simulink model "zadatak2"  (R2013b)
settings: Solver=ode45  StartTime=0.0  StopTime=10.0  RelTol=1e-3
settings Model: Creator=KORISNIK  LastModifiedBy=KORISNIK

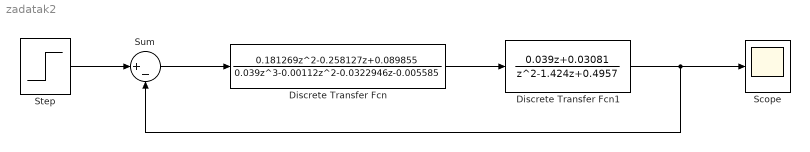
== system zadatak2 ==
  Discrete Transfer Fcn : DiscreteTransferFcn  Numerator=[0.181269 -0.258127 0.089855]  Denominator=[0.039 -0.00112 -0.0322946 -0.005585]  SampleTime=0.1
  Discrete Transfer Fcn1 : DiscreteTransferFcn  Numerator=[0.039 0.03081]  Denominator=[1 -1.424 0.4957]  SampleTime=0.1
  Scope : Scope
  Step : Step  SampleTime=0
  Sum : Sum  Inputs=|+-
  wires:
  Step/1 -> Sum/1
  Sum/1 -> Discrete Transfer Fcn/1
  Discrete Transfer Fcn/1 -> Discrete Transfer Fcn1/1
  Discrete Transfer Fcn1/1 -> Sum/2, Scope/1
